simulink model "l2"  (R2016a)
settings: Solver=ode23  StartTime=0.0  StopTime=100.0  RelTol=1e-3
libraries: simulink x1
settings Model: Creator=wojta  LastModifiedBy=wojta

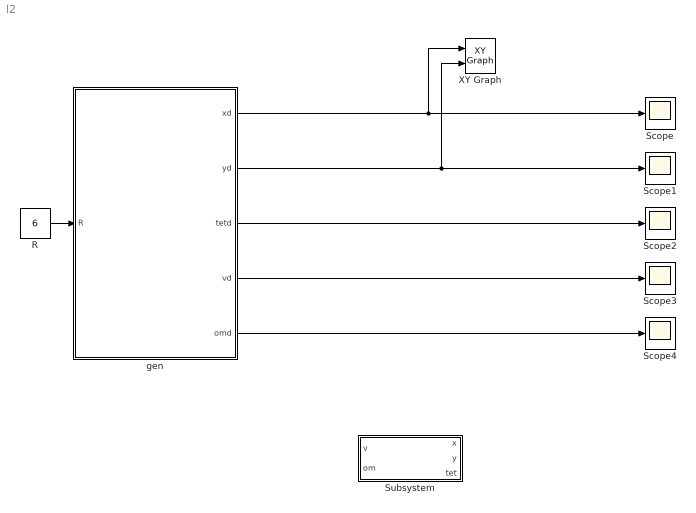
== system l2 ==
  R : Constant  Value=6
  Scope{,1..4} (5 alike) : Scope
  Subsystem : Subsystem
  XY Graph : simulink/Sinks/XY Graph  xmin=-7  xmax=7  ymin=-7  ymax=7  st=-1
  gen : Subsystem
  wires:
  R/1 -> gen/1(R)
  gen/1(xd) -> XY Graph/1, Scope/1
  gen/2(yd) -> XY Graph/2, Scope1/1
  gen/3(tetd) -> Scope2/1
  gen/4(vd) -> Scope3/1
  gen/5(omd) -> Scope4/1

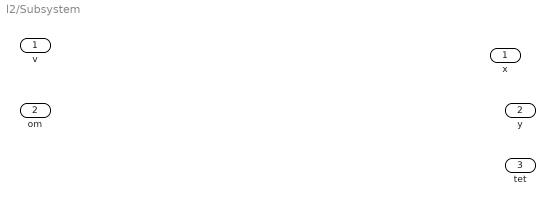
== system l2/Subsystem ==
  v : Inport
  om : Inport  Port=2
  x : Outport
  y : Outport  Port=2
  tet : Outport  Port=3

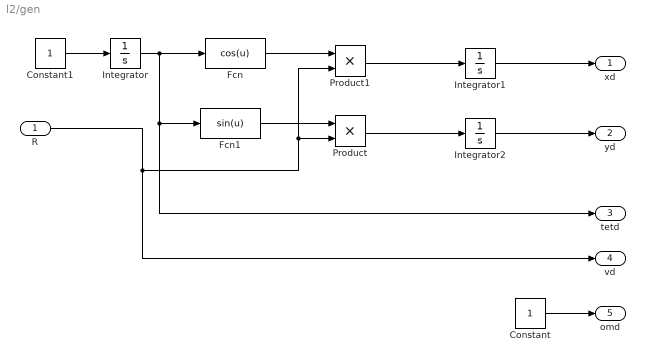
== system l2/gen ==
  R : Inport
  Constant : Constant
  Constant1 : Constant
  Fcn : Fcn  Expr=cos(u)
  Fcn1 : Fcn  Expr=sin(u)
  Integrator : Integrator
  Integrator1 : Integrator
  Integrator2 : Integrator  InitialCondition=-6
  Product : Product
  Product1 : Product
  xd : Outport
  yd : Outport  Port=2
  tetd : Outport  Port=3
  vd : Outport  Port=4
  omd : Outport  Port=5
  wires:
  Constant/1 -> omd/1
  R/1 -> Product1/2, Product/2, vd/1
  Constant1/1 -> Integrator/1
  Integrator/1 -> Fcn1/1, tetd/1, Fcn/1
  Fcn1/1 -> Product/1
  Fcn/1 -> Product1/1
  Product/1 -> Integrator2/1
  Product1/1 -> Integrator1/1
  Integrator1/1 -> xd/1
  Integrator2/1 -> yd/1
